simulink model "torque_controller_without_torque_loop_autotuner_final_version"  (R2020a)
settings: Solver=VariableStepAuto  StartTime=0.0  StopTime=5  RelTol=1e-3
model workspace (MAT data in the model file):
  DCBusVoltage = 24
  K_e = 221.0633
  L_d = 0.003482
  L_q = 0.00456
  Machine_Temperature = 25
  N = 9
  Peak_Current_String = 'Peak Current = 6.000000'
  PhaseAdvancesPerCycle = 36
  Phase_Advance_String = 'PhaseAdvance = 180.000000'
  PointsPerCycle = 36
  Rload = 1000000
  Rs = 0.624570538244
  Shaft_Speed = 27
  Sig : Simulink.Signal (value not decoded)
  Sig1 : Simulink.Signal (value not decoded)
  angleVec = [0 1.11111111111 2.22222222222 3.33333333333 4.44444444444 5.55555555556 6.66666666667 7.77777777778 8.88888888889 10 11.1111111111 12.2222222222 ... (37 elements, 1x37)]
  dq_inductance = 0.008366
  fluxAmat = [5.78758604472e-05 -0.00245230641441 -0.00496086974489 -0.00746825845512 -0.00997085180846 -0.0124701917234 -0.0149650380151 -0.0174527751443 -0.0199339133996 -0.0224017046643 -0.0248570910938 -0.0273006981398 ... (16428 elements, 12x37x37)]
  fluxD = 0.129208614948
  fluxDmat = [0.129332720835 0.129331856309 0.129330386347 0.129326055027 0.129320008491 0.129311398581 0.12929964601 0.129284600324 0.129267743431 0.129250546721 0.129230887735 0.129208614948 ... (16428 elements, 12x37x37)]
  fluxQ = -0.0273006981398
  fluxQmat = [5.78758604472e-05 -0.00245230641441 -0.00496086974489 -0.00746825845512 -0.00997085180846 -0.0124701917234 -0.0149650380151 -0.0174527751443 -0.0199339133996 -0.0224017046643 -0.0248570910938 -0.0273006981398 ... (16428 elements, 12x37x37)]
  fluxes = [-0.0273006981398; -0.0982475938625; 0.125548292002]
  funcresult = 0
  gammaVec = [-180 -170 -160 -150 -140 -130 -120 -110 -100 -90 -80 -70 ... (37 elements, 1x37)]
  i = 12
  invP = [-2.44929359829e-16  1; -0.866025403784  -0.5; 0.866025403784  -0.5]
  j = 37
  m = 37
  magVec = [0 0.545454545455 1.09090909091 1.63636363636 2.18181818182 2.72727272727 3.27272727273 3.81818181818 4.36363636364 4.90909090909 5.45454545455 6]
  mcad : handle (value not decoded)
  nGamma = 37
  nMag = 12
  nX = 37
  poleNumber = 18
  pole_pairs = 9
  res1 = 0
  res2 = 0
  res3 = 0
  resistance_per_phase = 0.6246
  simlog_MotorCAD_MATLAB_Simscape_Example : simscape.logging.Node (value not decoded)
  torque = -10.6713070894
  torqueMat = [-0.000127780443833 -0.972425785337 -1.94471415001 -2.91686171491 -3.8887574387 -4.86000619896 -5.83073162472 -6.80075888771 -7.77012767412 -8.7384579087 -9.70556312381 -10.6713070894 ... (16428 elements, 12x37x37)]
  torque_constant = 1.7505
  x1 = 360
  x2 = 360
  x3 = 360
  xe = 6.28318530718
  xlabel_string = 'Rotor angle (electrical °)'
  ylabel_string = 'Phase advance (°)'
libraries: fl_lib x13, nesl_utility x12, ee_lib x7, eeTransforms x3, slctrlblks x2, simulink x2, powerlib_meascontrol x1, powerlib x1
(part 2 of 2)

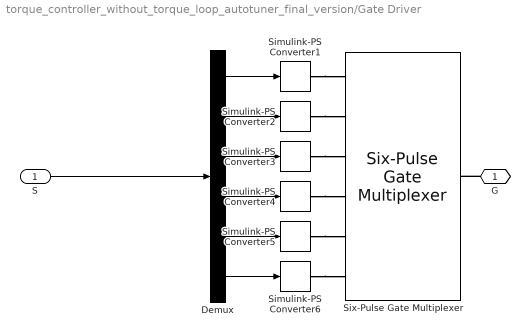
== system torque_controller_without_torque_loop_autotuner_final_version/Gate Driver ==
  S : Inport
  Demux : Demux  Outputs=6
  Simulink-PS Converter{1..6} (6 alike) : nesl_utility/Simulink-PS Converter  PhysicalDomain=network_engine_domain  SubClassName=ps_input  LeftPortType=input  RightPortType=output  PseudoPeriodic=off  Frequencies=[]  NoiseDistribution=none  NoiseParameters=[]  Unit=1  AffineConversion=off  FilteringAndDerivatives=zero  SimscapeFilterOrder=1  InputFilterTimeConstant=0.001  UdotUserProvided=1
      settings: SourceProductBaseCode=MT,SS
  Six-Pulse Gate Multiplexer : ee_lib/Semiconductors & Converters/Converters/Six-Pulse Gate Multiplexer  R=0 Ohm
      settings: SourceProductBaseCode=PS  InternalSimscapePortConfiguration="{\"Bottom\":[],\"Left\":[{\"id\":\"GaH\",\"label\":\"Ga(H)\",\"type\":\"input\"},{\"id\":\"GaL\",\"label\":\"Ga(L)\",\"type\":\"input\"},{\"id\":\"GbH\",\"label\":\"Gb(H)\",\"type\":\"input\"},{\"id\":\"GbL\",\"label\":\"Gb(L)\",\"type\":\"input\"},{\"id\":\"GcH\",\"label\":\"Gc(H)\",\"type\":\"input\"},{\"id\":\"GcL\",\"label\":\"Gc(L)\",\"type\":\"input\"}],\"Right\":[{\"id\":\"p\",\"label\":\"G\",\"type\":\"foundation.electrical.twelve_phase\"}],\"Top\":[]}"
  G : PMIOPort  Side=Right
  wires:
  Demux/1 -> Simulink-PS Converter1/1
  Demux/4 -> Simulink-PS Converter4/1
  Demux/2 -> Simulink-PS Converter2/1
  Demux/3 -> Simulink-PS Converter3/1
  Demux/5 -> Simulink-PS Converter5/1
  Demux/6 -> Simulink-PS Converter6/1
  S/1 -> Demux/1
  connections:
  G/RConn1 -- Six-Pulse Gate Multiplexer/RConn1
  Simulink-PS Converter5/RConn1 -- Six-Pulse Gate Multiplexer/LConn5
  Simulink-PS Converter4/RConn1 -- Six-Pulse Gate Multiplexer/LConn4
  Simulink-PS Converter6/RConn1 -- Six-Pulse Gate Multiplexer/LConn6
  Simulink-PS Converter3/RConn1 -- Six-Pulse Gate Multiplexer/LConn3
  Simulink-PS Converter2/RConn1 -- Six-Pulse Gate Multiplexer/LConn2
  Simulink-PS Converter1/RConn1 -- Six-Pulse Gate Multiplexer/LConn1

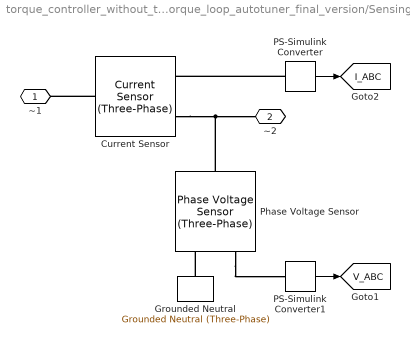
== system torque_controller_without_torque_loop_autotuner_final_version/Sensing vi ==
  Current Sensor : ee_lib/Sensors & Transducers/Current Sensor (Three-Phase)
  Grounded Neutral : ee_lib/Connectors & References/Grounded Neutral (Three-Phase)
      settings: SourceProductBaseCode=PS
  PS-Simulink Converter : nesl_utility/PS-Simulink Converter  PhysicalDomain=network_engine_domain  SubClassName=ps_output  LeftPortType=input  RightPortType=output  PseudoPeriodic=off  Frequencies=[]  Unit=A  AffineConversion=off
      settings: SourceProductBaseCode=MT,SS
  PS-Simulink Converter1 : nesl_utility/PS-Simulink Converter  PhysicalDomain=network_engine_domain  SubClassName=ps_output  LeftPortType=input  RightPortType=output  PseudoPeriodic=off  Frequencies=[]  Unit=V  AffineConversion=off
      settings: SourceProductBaseCode=MT,SS
  Phase Voltage Sensor : ee_lib/Sensors & Transducers/Phase Voltage Sensor (Three-Phase)
      settings: SourceProductBaseCode=PS
  ~1 : PMIOPort  Side=Left
  ~2 : PMIOPort  Port=2  Side=Right
  tag scope: I_ABC=global, V_ABC=global
  wires:
  PS-Simulink Converter/1 -> [I_ABC]
  PS-Simulink Converter1/1 -> [V_ABC]
  connections:
  Current Sensor/LConn1 -- ~1/RConn1
  PS-Simulink Converter/LConn1 -- Current Sensor/RConn1
  Current Sensor/RConn2 -- Phase Voltage Sensor/LConn1 -- ~2/RConn1
  Phase Voltage Sensor/RConn1 -- PS-Simulink Converter1/LConn1
  Grounded Neutral/LConn1 -- Phase Voltage Sensor/RConn2
